simulink model "IEEE14_case"  (R2024b)
settings: Solver=FixedStepAuto  StartTime=0  StopTime=2  FixedStep=1e-7  RelTol=1e-3
values from neighbouring files (symbols this model uses):
  GFL_15_Bva = 0.009    [IEEE14_parameters.m]
  GFL_15_C_bus_pu = 7.179419    [IEEE14_parameters.m]
  GFL_15_f0 = 60    [IEEE14_parameters.m]
  GFL_15_I_id = 691.26967    [IEEE14_parameters.m]
  GFL_15_I_iq = 691.26967    [IEEE14_parameters.m]
  GFL_15_I_od = 45.2207    [IEEE14_parameters.m]
  GFL_15_I_oq = 45.2207    [IEEE14_parameters.m]
  GFL_15_I_pll = 0.78    [IEEE14_parameters.m]
  GFL_15_Kdi = 0.09    [IEEE14_parameters.m]
  GFL_15_Kdo = 0.9    [IEEE14_parameters.m]
  GFL_15_Kqi = 0.09    [IEEE14_parameters.m]
  GFL_15_Kqo = 0.9    [IEEE14_parameters.m]
  GFL_15_Lg_pu = 0.631447    [IEEE14_parameters.m]
  GFL_15_mode = 1    [IEEE14_parameters.m]
  GFL_15_P_id = 3.7166    [IEEE14_parameters.m]
  GFL_15_P_iq = 3.7166    [IEEE14_parameters.m]
  GFL_15_P_od = 0.4798    [IEEE14_parameters.m]
  GFL_15_P_oq = 0.4798    [IEEE14_parameters.m]
  GFL_15_P_pll = 290.42    [IEEE14_parameters.m]
  GFL_15_Qe_ref = 0.2    [IEEE14_parameters.m]
  GFL_15_Rg_pu = 0.024016    [IEEE14_parameters.m]
  GFL_15_Sbase = 1.000000e+4    (= 10000)    [IEEE14_parameters.m]
  GFL_15_Tdi = 0.01    [IEEE14_parameters.m]
  GFL_15_Tdo = 0.2    [IEEE14_parameters.m]
  GFL_15_Tqi = 0.01    [IEEE14_parameters.m]
  GFL_15_Tqo = 0.2    [IEEE14_parameters.m]
  GFL_15_Vbase = 380    [IEEE14_parameters.m]
  GFL_15_Vdc_ref = 1.011475    [IEEE14_parameters.m]
  GFL_15_Vdcbase = 700    [IEEE14_parameters.m]
  GFL_15_vq_ref = 0    [IEEE14_parameters.m]
  GFL_16_Bva = 0.002    [IEEE14_parameters.m]
  GFL_16_C_bus_pu = 7.179419    [IEEE14_parameters.m]
  GFL_16_f0 = 60    [IEEE14_parameters.m]
  GFL_16_I_id = 691.26967    [IEEE14_parameters.m]
  GFL_16_I_iq = 691.26967    [IEEE14_parameters.m]
  GFL_16_I_od = 45.2207    [IEEE14_parameters.m]
  GFL_16_I_oq = 45.2207    [IEEE14_parameters.m]
  GFL_16_I_pll = 0.78    [IEEE14_parameters.m]
  GFL_16_Kdi = 0.05    [IEEE14_parameters.m]
  GFL_16_Kdo = 0.5    [IEEE14_parameters.m]
  GFL_16_Kqi = 0.05    [IEEE14_parameters.m]
  GFL_16_Kqo = 0.5    [IEEE14_parameters.m]
  GFL_16_Lg_pu = 0.631447    [IEEE14_parameters.m]
  GFL_16_mode = 1    [IEEE14_parameters.m]
  GFL_16_P_id = 3.7166    [IEEE14_parameters.m]
  GFL_16_P_iq = 3.7166    [IEEE14_parameters.m]
  GFL_16_P_od = 0.4798    [IEEE14_parameters.m]
  GFL_16_P_oq = 0.4798    [IEEE14_parameters.m]
  GFL_16_P_pll = 290.42    [IEEE14_parameters.m]
  GFL_16_Qe_ref = 0.2    [IEEE14_parameters.m]
  GFL_16_Rg_pu = 0.024016    [IEEE14_parameters.m]
  GFL_16_Sbase = 1.000000e+4    (= 10000)    [IEEE14_parameters.m]
  GFL_16_Tdi = 0.01    [IEEE14_parameters.m]
  GFL_16_Tdo = 0.2    [IEEE14_parameters.m]
  GFL_16_Tqi = 0.01    [IEEE14_parameters.m]
  GFL_16_Tqo = 0.2    [IEEE14_parameters.m]
  GFL_16_Vbase = 380    [IEEE14_parameters.m]
  GFL_16_Vdc_ref = 1.01144    [IEEE14_parameters.m]
  GFL_16_Vdcbase = 700    [IEEE14_parameters.m]
  GFL_16_vq_ref = 0    [IEEE14_parameters.m]
  GFL_17_Bva = 0.002    [IEEE14_parameters.m]
  GFL_17_C_bus_pu = 7.179419    [IEEE14_parameters.m]
  GFL_17_f0 = 60    [IEEE14_parameters.m]
  GFL_17_I_id = 691.26967    [IEEE14_parameters.m]
  GFL_17_I_iq = 691.26967    [IEEE14_parameters.m]
  GFL_17_I_od = 45.2207    [IEEE14_parameters.m]
  GFL_17_I_oq = 45.2207    [IEEE14_parameters.m]
  GFL_17_I_pll = 0.78    [IEEE14_parameters.m]
  GFL_17_Kdi = 0.05    [IEEE14_parameters.m]
  GFL_17_Kdo = 0.5    [IEEE14_parameters.m]
  GFL_17_Kqi = 0.05    [IEEE14_parameters.m]
  GFL_17_Kqo = 0.5    [IEEE14_parameters.m]
  GFL_17_Lg_pu = 0.631447    [IEEE14_parameters.m]
  GFL_17_mode = 1    [IEEE14_parameters.m]
  GFL_17_P_id = 3.7166    [IEEE14_parameters.m]
  GFL_17_P_iq = 3.7166    [IEEE14_parameters.m]
  GFL_17_P_od = 0.4798    [IEEE14_parameters.m]
  GFL_17_P_oq = 0.4798    [IEEE14_parameters.m]
  GFL_17_P_pll = 290.42    [IEEE14_parameters.m]
  GFL_17_Qe_ref = 0.2    [IEEE14_parameters.m]
  GFL_17_Rg_pu = 0.024016    [IEEE14_parameters.m]
  GFL_17_Sbase = 1.000000e+4    (= 10000)    [IEEE14_parameters.m]
  GFL_17_Tdi = 0.01    [IEEE14_parameters.m]
  GFL_17_Tdo = 0.2    [IEEE14_parameters.m]
  GFL_17_Tqi = 0.01    [IEEE14_parameters.m]
  GFL_17_Tqo = 0.2    [IEEE14_parameters.m]
  GFL_17_Vbase = 380    [IEEE14_parameters.m]
  GFL_17_Vdc_ref = 1.011632    [IEEE14_parameters.m]
  GFL_17_Vdcbase = 700    [IEEE14_parameters.m]
  GFL_17_vq_ref = 0    [IEEE14_parameters.m]
  GFL_18_Bva = 0.002    [IEEE14_parameters.m]
  GFL_18_C_bus_pu = 7.179419    [IEEE14_parameters.m]
  GFL_18_f0 = 60    [IEEE14_parameters.m]
  GFL_18_I_id = 691.26967    [IEEE14_parameters.m]
  GFL_18_I_iq = 691.26967    [IEEE14_parameters.m]
  GFL_18_I_od = 45.2207    [IEEE14_parameters.m]
  GFL_18_I_oq = 45.2207    [IEEE14_parameters.m]
  GFL_18_I_pll = 0.78    [IEEE14_parameters.m]
  GFL_18_Kdi = 0.05    [IEEE14_parameters.m]
  GFL_18_Kdo = 0.5    [IEEE14_parameters.m]
  GFL_18_Kqi = 0.05    [IEEE14_parameters.m]
  GFL_18_Kqo = 0.5    [IEEE14_parameters.m]
  GFL_18_Lg_pu = 0.631447    [IEEE14_parameters.m]
  GFL_18_mode = 1    [IEEE14_parameters.m]
  GFL_18_P_id = 3.7166    [IEEE14_parameters.m]
  GFL_18_P_iq = 3.7166    [IEEE14_parameters.m]
  GFL_18_P_od = 0.4798    [IEEE14_parameters.m]
  GFL_18_P_oq = 0.4798    [IEEE14_parameters.m]
  GFL_18_P_pll = 290.42    [IEEE14_parameters.m]
  GFL_18_Qe_ref = 0.2    [IEEE14_parameters.m]
  GFL_18_Rg_pu = 0.024016    [IEEE14_parameters.m]
  GFL_18_Sbase = 1.000000e+4    (= 10000)    [IEEE14_parameters.m]
  GFL_18_Tdi = 0.01    [IEEE14_parameters.m]
  GFL_18_Tdo = 0.2    [IEEE14_parameters.m]
  GFL_18_Tqi = 0.01    [IEEE14_parameters.m]
  GFL_18_Tqo = 0.2    [IEEE14_parameters.m]
  GFL_18_Vbase = 380    [IEEE14_parameters.m]
  GFL_18_Vdc_ref = 1.011572    [IEEE14_parameters.m]
  GFL_18_Vdcbase = 700    [IEEE14_parameters.m]
  GFL_18_vq_ref = 0    [IEEE14_parameters.m]
  ... (+180 more)
(part 5 of 25)

== system IEEE14_case/SG_D_8 ==
  v_d_SG_D_8 : Inport
  v_q_SG_D_8 : Inport  Port=2
  E_fd_SG_D_8 : Integrator  InitialCondition=0.7606400090631968
  Px_1_SG_D_8 : Integrator  InitialCondition=0.0
  Px_2_SG_D_8 : Integrator  InitialCondition=0.0
  Px_3_SG_D_8 : Integrator  InitialCondition=-4.623242258888885e-24
  R_f_SG_D_8 : Integrator  InitialCondition=5.135406689760955
  T_e_SG_D_8_block : Subsystem
  T_m_SG_D_8 : Integrator  InitialCondition=3.269365263487632e-05
  V_f_SG_D_8 : Integrator  InitialCondition=7.606400090631968
  d_E_fd_SG_D_8_block : Subsystem
  d_Px_1_SG_D_8_block : Subsystem
  d_Px_2_SG_D_8_block : Subsystem
  d_Px_3_SG_D_8_block : Subsystem
  d_R_f_SG_D_8_block : Subsystem
  d_T_m_SG_D_8_block : Subsystem
  d_V_f_SG_D_8_block : Subsystem
  d_psi_1d_SG_D_8_block : Subsystem
  d_psi_d_SG_D_8_block : Subsystem
  d_psi_fd_SG_D_8_block : Subsystem
  d_psi_gq_SG_D_8_block : Subsystem
  d_psi_kq_SG_D_8_block : Subsystem
  d_psi_q_SG_D_8_block : Subsystem
  d_theta_SG_D_8_block : Subsystem
  d_w_SG_D_8_block : Subsystem
  i_d_SG_D_8_block : Subsystem
  i_q_SG_D_8_block : Subsystem
  psi_1d_SG_D_8 : Integrator  InitialCondition=1.08133264662511
  psi_d_SG_D_8 : Integrator  InitialCondition=1.0900000152078642
  psi_fd_SG_D_8 : Integrator  InitialCondition=1.0376491089680278
  psi_gq_SG_D_8 : Integrator  InitialCondition=3.0249198689621347e-05
  psi_kq_SG_D_8 : Integrator  InitialCondition=-4.726437295253334e-05
  psi_q_SG_D_8 : Integrator  InitialCondition=-4.9154947870634654e-05
  theta_SG_D_8 : Integrator  InitialCondition=-0.18629255619094007
  theta_SG_D_8_out_block : Subsystem
  w_SG_D_8 : Integrator  InitialCondition=376.99111843077515
  w_SG_D_8_out_block : Subsystem
  i_d_SG_D_8 : Outport
  i_q_SG_D_8 : Outport  Port=2
  T_e_SG_D_8 : Outport  Port=3
  w_SG_D_8_out : Outport  Port=4
  theta_SG_D_8_out : Outport  Port=5
  wires:
  d_T_m_SG_D_8_block/1(Blockout_d_T_m_SG_D_8_65767) -> T_m_SG_D_8/1
  T_e_SG_D_8_block/1(Blockout_T_e_SG_D_8_36eef) -> T_e_SG_D_8/1
  theta_SG_D_8/1 -> d_psi_d_SG_D_8_block/5(State_theta_SG_D_8_aea71), d_psi_q_SG_D_8_block/5(State_theta_SG_D_8_01782), i_d_SG_D_8_block/4(State_theta_SG_D_8_641e8), i_d_SG_D_8_block/8(State_theta_SG_D_8_bcf58), d_psi_q_SG_D_8_block/7(State_theta_SG_D_8_5a3fa), i_q_SG_D_8_block/8(State_theta_SG_D_8_83255), d_psi_d_SG_D_8_block/7(State_theta_SG_D_8_9f713), theta_SG_D_8_out_block/1(State_theta_SG_D_8_cdb63), i_q_SG_D_8_block/4(State_theta_SG_D_8_df609)
  w_SG_D_8/1 -> d_psi_d_SG_D_8_block/9(State_w_SG_D_8_03911), d_psi_q_SG_D_8_block/9(State_w_SG_D_8_716c2), d_w_SG_D_8_block/1(State_w_SG_D_8_a443d), d_V_f_SG_D_8_block/8(State_w_SG_D_8_6dc7e), d_T_m_SG_D_8_block/1(State_w_SG_D_8_04413), d_theta_SG_D_8_block/1(State_w_SG_D_8_7874c), d_V_f_SG_D_8_block/13(State_w_SG_D_8_608f6), d_Px_2_SG_D_8_block/4(State_w_SG_D_8_213d1), d_Px_3_SG_D_8_block/6(State_w_SG_D_8_deb3f), w_SG_D_8_out_block/1(State_w_SG_D_8_62717), d_Px_1_SG_D_8_block/2(State_w_SG_D_8_14513)
  d_Px_2_SG_D_8_block/1(Blockout_d_Px_2_SG_D_8_ad385) -> Px_2_SG_D_8/1
  E_fd_SG_D_8/1 -> d_V_f_SG_D_8_block/1(State_E_fd_SG_D_8_0863f), d_E_fd_SG_D_8_block/1(State_E_fd_SG_D_8_6df86), d_R_f_SG_D_8_block/1(State_E_fd_SG_D_8_d418e), d_psi_fd_SG_D_8_block/1(State_E_fd_SG_D_8_e02cf)
  R_f_SG_D_8/1 -> d_V_f_SG_D_8_block/2(State_R_f_SG_D_8_6736f), d_R_f_SG_D_8_block/2(State_R_f_SG_D_8_19ab3)
  d_R_f_SG_D_8_block/1(Blockout_d_R_f_SG_D_8_431b8) -> R_f_SG_D_8/1
  w_SG_D_8_out_block/1(Blockout_w_SG_D_8_out_d72e6) -> w_SG_D_8_out/1
  d_Px_1_SG_D_8_block/1(Blockout_d_Px_1_SG_D_8_010b5) -> Px_1_SG_D_8/1
  d_theta_SG_D_8_block/1(Blockout_d_theta_SG_D_8_7fdd6) -> theta_SG_D_8/1
  d_Px_3_SG_D_8_block/1(Blockout_d_Px_3_SG_D_8_b7d57) -> Px_3_SG_D_8/1
  psi_gq_SG_D_8/1 -> d_psi_q_SG_D_8_block/1(State_psi_gq_SG_D_8_a7fd3), d_psi_gq_SG_D_8_block/1(State_psi_gq_SG_D_8_21c0a), d_psi_gq_SG_D_8_block/2(State_psi_gq_SG_D_8_953e4), d_psi_gq_SG_D_8_block/7(State_psi_gq_SG_D_8_869cf), d_psi_kq_SG_D_8_block/1(State_psi_gq_SG_D_8_46c2d), d_psi_kq_SG_D_8_block/3(State_psi_gq_SG_D_8_4cdf1), d_w_SG_D_8_block/4(State_psi_gq_SG_D_8_6cde6), i_d_SG_D_8_block/1(State_psi_gq_SG_D_8_6ad23), i_q_SG_D_8_block/1(State_psi_gq_SG_D_8_d57d0), d_V_f_SG_D_8_block/9(State_psi_gq_SG_D_8_341db), T_e_SG_D_8_block/2(State_psi_gq_SG_D_8_ece9e), d_psi_gq_SG_D_8_block/4(State_psi_gq_SG_D_8_d7d68)
  T_m_SG_D_8/1 -> d_T_m_SG_D_8_block/2(State_T_m_SG_D_8_6d384), d_w_SG_D_8_block/2(State_T_m_SG_D_8_49ad0)
  psi_q_SG_D_8/1 -> d_psi_d_SG_D_8_block/8(State_psi_q_SG_D_8_b70d1), d_psi_q_SG_D_8_block/3(State_psi_q_SG_D_8_e0430), d_psi_gq_SG_D_8_block/6(State_psi_q_SG_D_8_5d8c1), d_psi_gq_SG_D_8_block/9(State_psi_q_SG_D_8_ecb47), d_psi_kq_SG_D_8_block/5(State_psi_q_SG_D_8_6f170), d_w_SG_D_8_block/6(State_psi_q_SG_D_8_202ce), d_w_SG_D_8_block/7(State_psi_q_SG_D_8_9c5c1), d_V_f_SG_D_8_block/11(State_psi_q_SG_D_8_d5d6d), i_q_SG_D_8_block/3(State_psi_q_SG_D_8_a812b), i_d_SG_D_8_block/3(State_psi_q_SG_D_8_2ca29), T_e_SG_D_8_block/4(State_psi_q_SG_D_8_1c36c), d_V_f_SG_D_8_block/7(State_psi_q_SG_D_8_e1efb), T_e_SG_D_8_block/5(State_psi_q_SG_D_8_67075)
  Px_2_SG_D_8/1 -> d_Px_2_SG_D_8_block/1(State_Px_2_SG_D_8_4dc99), d_Px_3_SG_D_8_block/2(State_Px_2_SG_D_8_f1029), d_Px_3_SG_D_8_block/3(State_Px_2_SG_D_8_bb5ac)
  Px_3_SG_D_8/1 -> d_Px_3_SG_D_8_block/1(State_Px_3_SG_D_8_df285), d_V_f_SG_D_8_block/3(State_Px_3_SG_D_8_1b788)
  v_d_SG_D_8/1 -> d_psi_d_SG_D_8_block/4(Input_v_d_SG_D_8_41885), d_psi_q_SG_D_8_block/4(Input_v_d_SG_D_8_c09e8)
  d_psi_gq_SG_D_8_block/1(Blockout_d_psi_gq_SG_D_8_03a58) -> psi_gq_SG_D_8/1
  v_q_SG_D_8/1 -> d_psi_d_SG_D_8_block/6(Input_v_q_SG_D_8_e5b6f), d_psi_q_SG_D_8_block/6(Input_v_q_SG_D_8_1ed15)
  d_psi_1d_SG_D_8_block/1(Blockout_d_psi_1d_SG_D_8_20ff0) -> psi_1d_SG_D_8/1
  psi_fd_SG_D_8/1 -> d_psi_fd_SG_D_8_block/2(State_psi_fd_SG_D_8_39b4d), d_psi_fd_SG_D_8_block/4(State_psi_fd_SG_D_8_1b7c8), d_psi_fd_SG_D_8_block/7(State_psi_fd_SG_D_8_ed057), d_psi_fd_SG_D_8_block/10(State_psi_fd_SG_D_8_f6f0f), d_psi_d_SG_D_8_block/3(State_psi_fd_SG_D_8_f0d2e), d_psi_1d_SG_D_8_block/5(State_psi_fd_SG_D_8_c65e7), d_w_SG_D_8_block/10(State_psi_fd_SG_D_8_93d32), d_psi_1d_SG_D_8_block/2(State_psi_fd_SG_D_8_4604f), i_d_SG_D_8_block/7(State_psi_fd_SG_D_8_06311), i_q_SG_D_8_block/7(State_psi_fd_SG_D_8_e7c26), d_V_f_SG_D_8_block/6(State_psi_fd_SG_D_8_8705e), T_e_SG_D_8_block/8(State_psi_fd_SG_D_8_0a0bc)
  psi_1d_SG_D_8/1 -> d_psi_fd_SG_D_8_block/3(State_psi_1d_SG_D_8_31c78), d_psi_fd_SG_D_8_block/5(State_psi_1d_SG_D_8_9e1bf), d_psi_fd_SG_D_8_block/8(State_psi_1d_SG_D_8_5095e), d_psi_d_SG_D_8_block/1(State_psi_1d_SG_D_8_3a1ac), d_psi_1d_SG_D_8_block/3(State_psi_1d_SG_D_8_0fd5c), i_d_SG_D_8_block/5(State_psi_1d_SG_D_8_b3820), i_q_SG_D_8_block/5(State_psi_1d_SG_D_8_47e6f), T_e_SG_D_8_block/6(State_psi_1d_SG_D_8_d92c8), d_V_f_SG_D_8_block/4(State_psi_1d_SG_D_8_0200e), d_psi_1d_SG_D_8_block/1(State_psi_1d_SG_D_8_961b1), d_w_SG_D_8_block/8(State_psi_1d_SG_D_8_25d54)
  psi_d_SG_D_8/1 -> d_psi_fd_SG_D_8_block/6(State_psi_d_SG_D_8_43284), d_psi_fd_SG_D_8_block/9(State_psi_d_SG_D_8_8f483), d_psi_d_SG_D_8_block/2(State_psi_d_SG_D_8_aedd8), d_psi_1d_SG_D_8_block/4(State_psi_d_SG_D_8_df1ee), d_w_SG_D_8_block/3(State_psi_d_SG_D_8_19a89), d_w_SG_D_8_block/9(State_psi_d_SG_D_8_5f3fa), d_V_f_SG_D_8_block/5(State_psi_d_SG_D_8_c5413), d_V_f_SG_D_8_block/12(State_psi_d_SG_D_8_14bfc), i_d_SG_D_8_block/6(State_psi_d_SG_D_8_f7e33), i_q_SG_D_8_block/6(State_psi_d_SG_D_8_17299), T_e_SG_D_8_block/7(State_psi_d_SG_D_8_41989), d_psi_q_SG_D_8_block/8(State_psi_d_SG_D_8_332cc), T_e_SG_D_8_block/1(State_psi_d_SG_D_8_8bce2)
  psi_kq_SG_D_8/1 -> d_psi_q_SG_D_8_block/2(State_psi_kq_SG_D_8_644c1), d_psi_gq_SG_D_8_block/3(State_psi_kq_SG_D_8_6a8ed), d_psi_gq_SG_D_8_block/5(State_psi_kq_SG_D_8_1ecc5), d_psi_kq_SG_D_8_block/2(State_psi_kq_SG_D_8_36a8a), d_psi_gq_SG_D_8_block/8(State_psi_kq_SG_D_8_7be32), d_psi_kq_SG_D_8_block/4(State_psi_kq_SG_D_8_90e06), i_d_SG_D_8_block/2(State_psi_kq_SG_D_8_4cd34), d_w_SG_D_8_block/5(State_psi_kq_SG_D_8_f145c), i_q_SG_D_8_block/2(State_psi_kq_SG_D_8_4aaa9), d_V_f_SG_D_8_block/10(State_psi_kq_SG_D_8_85c57), T_e_SG_D_8_block/3(State_psi_kq_SG_D_8_39808)
  Px_1_SG_D_8/1 -> d_Px_1_SG_D_8_block/1(State_Px_1_SG_D_8_6e138), d_Px_3_SG_D_8_block/4(State_Px_1_SG_D_8_7f9bd), d_Px_2_SG_D_8_block/3(State_Px_1_SG_D_8_35ac2), d_Px_2_SG_D_8_block/2(State_Px_1_SG_D_8_d499c), d_Px_3_SG_D_8_block/5(State_Px_1_SG_D_8_8b47e)
  d_w_SG_D_8_block/1(Blockout_d_w_SG_D_8_91fe0) -> w_SG_D_8/1
  d_psi_kq_SG_D_8_block/1(Blockout_d_psi_kq_SG_D_8_f1e70) -> psi_kq_SG_D_8/1
  d_V_f_SG_D_8_block/1(Blockout_d_V_f_SG_D_8_302ea) -> V_f_SG_D_8/1
  d_psi_q_SG_D_8_block/1(Blockout_d_psi_q_SG_D_8_90d0e) -> psi_q_SG_D_8/1
  d_psi_d_SG_D_8_block/1(Blockout_d_psi_d_SG_D_8_dc023) -> psi_d_SG_D_8/1
  i_q_SG_D_8_block/1(Blockout_i_q_SG_D_8_09699) -> i_q_SG_D_8/1
  i_d_SG_D_8_block/1(Blockout_i_d_SG_D_8_0f0f6) -> i_d_SG_D_8/1
  theta_SG_D_8_out_block/1(Blockout_theta_SG_D_8_out_2e6e5) -> theta_SG_D_8_out/1
  V_f_SG_D_8/1 -> d_V_f_SG_D_8_block/14(State_V_f_SG_D_8_f18fe), d_E_fd_SG_D_8_block/2(State_V_f_SG_D_8_2f3e7)
  d_E_fd_SG_D_8_block/1(Blockout_d_E_fd_SG_D_8_bd076) -> E_fd_SG_D_8/1
  d_psi_fd_SG_D_8_block/1(Blockout_d_psi_fd_SG_D_8_d8ca3) -> psi_fd_SG_D_8/1

== system IEEE14_case/Subsystem ==
  In1 : Inport
  In2 : Inport  Port=2
  In3 : Inport  Port=3
  In4 : Inport  Port=4
  Add : Sum
  Product : Product
  Product1 : Product
  Out1 : Outport
  wires:
  Product/1 -> Add/1
  In1/1 -> Product/1
  In3/1 -> Product1/1
  In2/1 -> Product/2
  Add/1 -> Out1/1
  Product1/1 -> Add/2
  In4/1 -> Product1/2

== system IEEE14_case/Subsystem1 ==
  In1 : Inport
  In2 : Inport  Port=2
  In3 : Inport  Port=3
  In4 : Inport  Port=4
  Add1 : Sum  Inputs=+-
  Product2 : Product
  Product3 : Product
  Out1 : Outport
  wires:
  In4/1 -> Product3/2
  Product3/1 -> Add1/2
  Product2/1 -> Add1/1
  In3/1 -> Product3/1
  In1/1 -> Product2/1
  Add1/1 -> Out1/1
  In2/1 -> Product2/2

== system IEEE14_case/AC_1/d_id_line_10_11_block ==
  note: d_id_line_10_11 in case14gfl
      | $376.991118430775\,\mathrm{iq}_{\mathrm{line},10,11}-161.046083548941\,\mathrm{id}_{\mathrm{line},10,11}+1962.77981168728\,\mathrm{vd}_{\mathrm{bus},10}-1962.77981168728\,\mathrm{vd}_{\mathrm{bus},11}$
      | Automatically generated on 2025-10-09 21:39:46 .
  State_id_line_10_11_cd03d : Inport
  State_iq_line_10_11_98837 : Inport  Port=2
  State_vd_bus_10_b9381 : Inport  Port=3
  State_vd_bus_11_0464d : Inport  Port=4
  Add_044af : Sum
  Add_952f4 : Sum
  Constant_-161.046083548941_02036 : Constant  Value=-161.046083548941
  Constant_1962.77981168728_222ef : Constant  Value=1962.77981168728
  Constant_1962.77981168728_ae5a8 : Constant  Value=1962.77981168728
  Constant_376.991118430775_6ba22 : Constant  Value=376.991118430775
  Product_7b56a : Product
  Product_7fb11 : Product
  Product_aa4a9 : Product
  Product_fe1f1 : Product
  Subtract_21330 : Sum  Inputs=+-
  Blockout_d_id_line_10_11_2eb24 : Outport
  wires:
  Constant_-161.046083548941_02036/1 -> Product_7b56a/1
  Subtract_21330/1 -> Blockout_d_id_line_10_11_2eb24/1
  State_id_line_10_11_cd03d/1 -> Product_7b56a/2
  Constant_376.991118430775_6ba22/1 -> Product_aa4a9/1
  Product_aa4a9/1 -> Add_044af/2
  Product_7fb11/1 -> Add_952f4/2
  Constant_1962.77981168728_222ef/1 -> Product_7fb11/1
  State_iq_line_10_11_98837/1 -> Product_aa4a9/2
  Product_7b56a/1 -> Add_044af/1
  State_vd_bus_10_b9381/1 -> Product_7fb11/2
  Add_044af/1 -> Add_952f4/1
  Product_fe1f1/1 -> Subtract_21330/2
  Constant_1962.77981168728_ae5a8/1 -> Product_fe1f1/1
  State_vd_bus_11_0464d/1 -> Product_fe1f1/2
  Add_952f4/1 -> Subtract_21330/1

== system IEEE14_case/AC_1/d_id_line_11_15_block ==
  note: d_id_line_11_15 in case14gfl
      | $376.991118430775\,\mathrm{iq}_{\mathrm{line},11,15}-32.3135244369236\,\mathrm{id}_{\mathrm{line},11,15}+538.558740615393\,\mathrm{vd}_{\mathrm{bus},11}-538.558740615393\,\mathrm{vd}_{\mathrm{bus},15}$
      | Automatically generated on 2025-10-09 21:39:53 .
  State_id_line_11_15_bc21e : Inport
  State_iq_line_11_15_e6608 : Inport  Port=2
  State_vd_bus_11_d33d1 : Inport  Port=3
  State_vd_bus_15_a703b : Inport  Port=4
  Add_9e7fa : Sum
  Add_ec072 : Sum
  Constant_-32.3135244369236_ce476 : Constant  Value=-32.3135244369236
  Constant_376.991118430775_cd329 : Constant  Value=376.991118430775
  Constant_538.558740615393_1f99f : Constant  Value=538.558740615393
  Constant_538.558740615393_64059 : Constant  Value=538.558740615393
  Product_5d9cb : Product
  Product_5fd59 : Product
  Product_c3b90 : Product
  Product_c9bc5 : Product
  Subtract_ad8a8 : Sum  Inputs=+-
  Blockout_d_id_line_11_15_7b448 : Outport
  wires:
  Constant_-32.3135244369236_ce476/1 -> Product_5d9cb/1
  Product_5d9cb/1 -> Add_ec072/1
  State_id_line_11_15_bc21e/1 -> Product_5d9cb/2
  Constant_376.991118430775_cd329/1 -> Product_c9bc5/1
  Product_c9bc5/1 -> Add_ec072/2
  State_iq_line_11_15_e6608/1 -> Product_c9bc5/2
  State_vd_bus_11_d33d1/1 -> Product_c3b90/2
  Product_c3b90/1 -> Add_9e7fa/2
  Constant_538.558740615393_64059/1 -> Product_c3b90/1
  Add_ec072/1 -> Add_9e7fa/1
  Product_5fd59/1 -> Subtract_ad8a8/2
  Constant_538.558740615393_1f99f/1 -> Product_5fd59/1
  Add_9e7fa/1 -> Subtract_ad8a8/1
  State_vd_bus_15_a703b/1 -> Product_5fd59/2
  Subtract_ad8a8/1 -> Blockout_d_id_line_11_15_7b448/1

== system IEEE14_case/AC_1/d_id_line_12_13_block ==
  note: d_id_line_12_13 in case14gfl
      | $376.991118430775\,\mathrm{iq}_{\mathrm{line},12,13}-416.674394055067\,\mathrm{id}_{\mathrm{line},12,13}+1886.08724450058\,\mathrm{vd}_{\mathrm{bus},12}-1886.08724450058\,\mathrm{vd}_{\mathrm{bus},13}$
      | Automatically generated on 2025-10-09 21:39:48 .
  State_id_line_12_13_dd6c1 : Inport
  State_iq_line_12_13_bd70b : Inport  Port=2
  State_vd_bus_12_5b3a8 : Inport  Port=3
  State_vd_bus_13_1a95e : Inport  Port=4
  Add_3f260 : Sum
  Add_fb038 : Sum
  Constant_-416.674394055067_9eb27 : Constant  Value=-416.674394055067
  Constant_1886.08724450058_572fc : Constant  Value=1886.08724450058
  Constant_1886.08724450058_d19a4 : Constant  Value=1886.08724450058
  Constant_376.991118430775_8657a : Constant  Value=376.991118430775
  Product_08de4 : Product
  Product_09161 : Product
  Product_3ee40 : Product
  Product_c6c0f : Product
  Subtract_69e56 : Sum  Inputs=+-
  Blockout_d_id_line_12_13_a63f9 : Outport
  wires:
  State_iq_line_12_13_bd70b/1 -> Product_3ee40/2
  Constant_-416.674394055067_9eb27/1 -> Product_08de4/1
  Constant_376.991118430775_8657a/1 -> Product_3ee40/1
  Product_3ee40/1 -> Add_fb038/2
  State_id_line_12_13_dd6c1/1 -> Product_08de4/2
  Product_08de4/1 -> Add_fb038/1
  Constant_1886.08724450058_d19a4/1 -> Product_09161/1
  State_vd_bus_12_5b3a8/1 -> Product_09161/2
  Add_fb038/1 -> Add_3f260/1
  Product_09161/1 -> Add_3f260/2
  Product_c6c0f/1 -> Subtract_69e56/2
  Constant_1886.08724450058_572fc/1 -> Product_c6c0f/1
  State_vd_bus_13_1a95e/1 -> Product_c6c0f/2
  Add_3f260/1 -> Subtract_69e56/1
  Subtract_69e56/1 -> Blockout_d_id_line_12_13_a63f9/1

== system IEEE14_case/AC_1/d_id_line_12_16_block ==
  note: d_id_line_12_16 in case14gfl
      | $376.991118430775\,\mathrm{iq}_{\mathrm{line},12,16}-32.3135244369236\,\mathrm{id}_{\mathrm{line},12,16}+538.558740615393\,\mathrm{vd}_{\mathrm{bus},12}-538.558740615393\,\mathrm{vd}_{\mathrm{bus},16}$
      | Automatically generated on 2025-10-09 21:39:55 .
  State_id_line_12_16_7c285 : Inport
  State_iq_line_12_16_b3649 : Inport  Port=2
  State_vd_bus_12_7f21e : Inport  Port=3
  State_vd_bus_16_b2ca7 : Inport  Port=4
  Add_71088 : Sum
  Add_cefde : Sum
  Constant_-32.3135244369236_989f2 : Constant  Value=-32.3135244369236
  Constant_376.991118430775_4638c : Constant  Value=376.991118430775
  Constant_538.558740615393_259c1 : Constant  Value=538.558740615393
  Constant_538.558740615393_4455a : Constant  Value=538.558740615393
  Product_4a5f5 : Product
  Product_8747e : Product
  Product_c16a2 : Product
  Product_f3dc0 : Product
  Subtract_95055 : Sum  Inputs=+-
  Blockout_d_id_line_12_16_c0fbf : Outport
  wires:
  State_id_line_12_16_7c285/1 -> Product_8747e/2
  Constant_-32.3135244369236_989f2/1 -> Product_8747e/1
  Constant_376.991118430775_4638c/1 -> Product_4a5f5/1
  Product_4a5f5/1 -> Add_71088/2
  Product_c16a2/1 -> Add_cefde/2
  Constant_538.558740615393_259c1/1 -> Product_c16a2/1
  State_iq_line_12_16_b3649/1 -> Product_4a5f5/2
  Product_8747e/1 -> Add_71088/1
  State_vd_bus_12_7f21e/1 -> Product_c16a2/2
  Add_71088/1 -> Add_cefde/1
  Product_f3dc0/1 -> Subtract_95055/2
  Constant_538.558740615393_4455a/1 -> Product_f3dc0/1
  State_vd_bus_16_b2ca7/1 -> Product_f3dc0/2
  Add_cefde/1 -> Subtract_95055/1
  Subtract_95055/1 -> Blockout_d_id_line_12_16_c0fbf/1

== system IEEE14_case/AC_1/d_id_line_13_14_block ==
  note: d_id_line_13_14 in case14gfl
      | $376.991118430775\,\mathrm{iq}_{\mathrm{line},13,14}-185.159162902627\,\mathrm{id}_{\mathrm{line},13,14}+1083.24555609096\,\mathrm{vd}_{\mathrm{bus},13}-1083.24555609096\,\mathrm{vd}_{\mathrm{bus},14}$
      | Automatically generated on 2025-10-09 21:39:50 .
  State_id_line_13_14_79a4b : Inport
  State_iq_line_13_14_4cdf7 : Inport  Port=2
  State_vd_bus_13_a4a43 : Inport  Port=3
  State_vd_bus_14_db328 : Inport  Port=4
  Add_2b3ae : Sum
  Add_92208 : Sum
  Constant_-185.159162902627_131b7 : Constant  Value=-185.159162902627
  Constant_1083.24555609096_5a0e7 : Constant  Value=1083.24555609096
  Constant_1083.24555609096_8e61e : Constant  Value=1083.24555609096
  Constant_376.991118430775_13321 : Constant  Value=376.991118430775
  Product_45268 : Product
  Product_c11f5 : Product
  Product_da29c : Product
  Product_f0334 : Product
  Subtract_95086 : Sum  Inputs=+-
  Blockout_d_id_line_13_14_fab77 : Outport
  wires:
  Constant_-185.159162902627_131b7/1 -> Product_45268/1
  Product_45268/1 -> Add_2b3ae/1
  Subtract_95086/1 -> Blockout_d_id_line_13_14_fab77/1
  State_id_line_13_14_79a4b/1 -> Product_45268/2
  Constant_376.991118430775_13321/1 -> Product_c11f5/1
  Product_c11f5/1 -> Add_2b3ae/2
  State_iq_line_13_14_4cdf7/1 -> Product_c11f5/2
  Product_f0334/1 -> Add_92208/2
  Constant_1083.24555609096_8e61e/1 -> Product_f0334/1
  State_vd_bus_13_a4a43/1 -> Product_f0334/2
  Add_2b3ae/1 -> Add_92208/1
  Constant_1083.24555609096_5a0e7/1 -> Product_da29c/1
  State_vd_bus_14_db328/1 -> Product_da29c/2
  Add_92208/1 -> Subtract_95086/1
  Product_da29c/1 -> Subtract_95086/2

== system IEEE14_case/AC_1/d_id_line_13_17_block ==
  note: d_id_line_13_17 in case14gfl
      | $376.991118430775\,\mathrm{iq}_{\mathrm{line},13,17}-32.3135244369236\,\mathrm{id}_{\mathrm{line},13,17}+538.558740615393\,\mathrm{vd}_{\mathrm{bus},13}-538.558740615393\,\mathrm{vd}_{\mathrm{bus},17}$
      | Automatically generated on 2025-10-09 21:39:57 .
  State_id_line_13_17_86061 : Inport
  State_iq_line_13_17_a0741 : Inport  Port=2
  State_vd_bus_13_e5c14 : Inport  Port=3
  State_vd_bus_17_94433 : Inport  Port=4
  Add_85017 : Sum
  Add_b41df : Sum
  Constant_-32.3135244369236_c0773 : Constant  Value=-32.3135244369236
  Constant_376.991118430775_c840a : Constant  Value=376.991118430775
  Constant_538.558740615393_15349 : Constant  Value=538.558740615393
  Constant_538.558740615393_4ce18 : Constant  Value=538.558740615393
  Product_17a6a : Product
  Product_257da : Product
  Product_a0416 : Product
  Product_e7a08 : Product
  Subtract_3675c : Sum  Inputs=+-
  Blockout_d_id_line_13_17_24730 : Outport
  wires:
  State_iq_line_13_17_a0741/1 -> Product_a0416/2
  Constant_-32.3135244369236_c0773/1 -> Product_e7a08/1
  Constant_376.991118430775_c840a/1 -> Product_a0416/1
  Product_a0416/1 -> Add_85017/2
  State_id_line_13_17_86061/1 -> Product_e7a08/2
  Product_e7a08/1 -> Add_85017/1
  Constant_538.558740615393_4ce18/1 -> Product_257da/1
  State_vd_bus_13_e5c14/1 -> Product_257da/2
  Add_85017/1 -> Add_b41df/1
  Product_257da/1 -> Add_b41df/2
  Product_17a6a/1 -> Subtract_3675c/2
  Constant_538.558740615393_15349/1 -> Product_17a6a/1
  State_vd_bus_17_94433/1 -> Product_17a6a/2
  Add_b41df/1 -> Subtract_3675c/1
  Subtract_3675c/1 -> Blockout_d_id_line_13_17_24730/1

== system IEEE14_case/AC_1/d_id_line_14_18_block ==
  note: d_id_line_14_18 in case14gfl
      | $376.991118430775\,\mathrm{iq}_{\mathrm{line},14,18}-32.3135244369236\,\mathrm{id}_{\mathrm{line},14,18}+538.558740615393\,\mathrm{vd}_{\mathrm{bus},14}-538.558740615393\,\mathrm{vd}_{\mathrm{bus},18}$
      | Automatically generated on 2025-10-09 21:40:00 .
  State_id_line_14_18_fb6d6 : Inport
  State_iq_line_14_18_a74d0 : Inport  Port=2
  State_vd_bus_14_f98b2 : Inport  Port=3
  State_vd_bus_18_b444f : Inport  Port=4
  Add_15b48 : Sum
  Add_7e766 : Sum
  Constant_-32.3135244369236_f6a71 : Constant  Value=-32.3135244369236
  Constant_376.991118430775_92094 : Constant  Value=376.991118430775
  Constant_538.558740615393_c6265 : Constant  Value=538.558740615393
  Constant_538.558740615393_d688d : Constant  Value=538.558740615393
  Product_0bcce : Product
  Product_44810 : Product
  Product_4ac6d : Product
  Product_99de6 : Product
  Subtract_b7c2c : Sum  Inputs=+-
  Blockout_d_id_line_14_18_3e263 : Outport
  wires:
  Constant_-32.3135244369236_f6a71/1 -> Product_99de6/1
  Product_99de6/1 -> Add_15b48/1
  State_id_line_14_18_fb6d6/1 -> Product_99de6/2
  Constant_376.991118430775_92094/1 -> Product_4ac6d/1
  Product_4ac6d/1 -> Add_15b48/2
  State_iq_line_14_18_a74d0/1 -> Product_4ac6d/2
  Product_0bcce/1 -> Add_7e766/2
  Constant_538.558740615393_c6265/1 -> Product_0bcce/1
  State_vd_bus_14_f98b2/1 -> Product_0bcce/2
  Add_15b48/1 -> Add_7e766/1
  Constant_538.558740615393_d688d/1 -> Product_44810/1
  State_vd_bus_18_b444f/1 -> Product_44810/2
  Add_7e766/1 -> Subtract_b7c2c/1
  Product_44810/1 -> Subtract_b7c2c/2
  Subtract_b7c2c/1 -> Blockout_d_id_line_14_18_3e263/1

== system IEEE14_case/AC_1/d_id_line_1_2_block ==
  note: d_id_line_1_2 in case14gfl
      | $376.991118430775\,\mathrm{iq}_{\mathrm{line},1,2}-123.476218948596\,\mathrm{id}_{\mathrm{line},1,2}+6371.32192717213\,\mathrm{vd}_{\mathrm{bus},1}-6371.32192717213\,\mathrm{vd}_{\mathrm{bus},2}$
      | Automatically generated on 2025-10-09 21:39:11 .
  State_id_line_1_2_4e64f : Inport
  State_iq_line_1_2_aada7 : Inport  Port=2
  State_vd_bus_1_70d37 : Inport  Port=3
  State_vd_bus_2_c09e1 : Inport  Port=4
  Add_a1930 : Sum
  Add_e754f : Sum
  Constant_-123.476218948596_5bf1b : Constant  Value=-123.476218948596
  Constant_376.991118430775_40784 : Constant  Value=376.991118430775
  Constant_6371.32192717213_38569 : Constant  Value=6371.32192717213
  Constant_6371.32192717213_e91b8 : Constant  Value=6371.32192717213
  Product_2be0d : Product
  Product_33e9b : Product
  Product_7e726 : Product
  Product_85465 : Product
  Subtract_08e95 : Sum  Inputs=+-
  Blockout_d_id_line_1_2_e6d8f : Outport
  wires:
  Constant_-123.476218948596_5bf1b/1 -> Product_2be0d/1
  Product_2be0d/1 -> Add_e754f/1
  State_id_line_1_2_4e64f/1 -> Product_2be0d/2
  Add_a1930/1 -> Subtract_08e95/1
  Constant_376.991118430775_40784/1 -> Product_33e9b/1
  Product_33e9b/1 -> Add_e754f/2
  State_iq_line_1_2_aada7/1 -> Product_33e9b/2
  Product_7e726/1 -> Add_a1930/2
  Constant_6371.32192717213_38569/1 -> Product_7e726/1
  Subtract_08e95/1 -> Blockout_d_id_line_1_2_e6d8f/1
  State_vd_bus_1_70d37/1 -> Product_7e726/2
  Add_e754f/1 -> Add_a1930/1
  Product_85465/1 -> Subtract_08e95/2
  Constant_6371.32192717213_e91b8/1 -> Product_85465/1
  State_vd_bus_2_c09e1/1 -> Product_85465/2

== system IEEE14_case/AC_1/d_id_line_1_5_block ==
  note: d_id_line_1_5 in case14gfl
      | $376.991118430775\,\mathrm{iq}_{\mathrm{line},1,5}-91.3236644943274\,\mathrm{id}_{\mathrm{line},1,5}+1690.23994992277\,\mathrm{vd}_{\mathrm{bus},1}-1690.23994992277\,\mathrm{vd}_{\mathrm{bus},5}$
      | Automatically generated on 2025-10-09 21:39:13 .
  State_id_line_1_5_7d5d3 : Inport
  State_iq_line_1_5_368c4 : Inport  Port=2
  State_vd_bus_1_768e4 : Inport  Port=3
  State_vd_bus_5_58650 : Inport  Port=4
  Add_8fb67 : Sum
  Add_b211a : Sum
  Constant_-91.3236644943274_4a822 : Constant  Value=-91.3236644943274
  Constant_1690.23994992277_5f559 : Constant  Value=1690.23994992277
  Constant_1690.23994992277_87596 : Constant  Value=1690.23994992277
  Constant_376.991118430775_d449f : Constant  Value=376.991118430775
  Product_0e523 : Product
  Product_275fb : Product
  Product_4af4f : Product
  Product_fdc0d : Product
  Subtract_4765f : Sum  Inputs=+-
  Blockout_d_id_line_1_5_95dd5 : Outport
  wires:
  Constant_-91.3236644943274_4a822/1 -> Product_0e523/1
  State_id_line_1_5_7d5d3/1 -> Product_0e523/2
  Constant_376.991118430775_d449f/1 -> Product_275fb/1
  Product_275fb/1 -> Add_b211a/2
  State_iq_line_1_5_368c4/1 -> Product_275fb/2
  Product_0e523/1 -> Add_b211a/1
  Constant_1690.23994992277_5f559/1 -> Product_4af4f/1
  State_vd_bus_1_768e4/1 -> Product_4af4f/2
  Add_b211a/1 -> Add_8fb67/1
  Product_4af4f/1 -> Add_8fb67/2
  Product_fdc0d/1 -> Subtract_4765f/2
  Constant_1690.23994992277_87596/1 -> Product_fdc0d/1
  State_vd_bus_5_58650/1 -> Product_fdc0d/2
  Add_8fb67/1 -> Subtract_4765f/1
  Subtract_4765f/1 -> Blockout_d_id_line_1_5_95dd5/1

== system IEEE14_case/AC_1/d_id_line_2_3_block ==
  note: d_id_line_2_3 in case14gfl
      | $376.991118430775\,\mathrm{iq}_{\mathrm{line},2,3}-89.482308708704\,\mathrm{id}_{\mathrm{line},2,3}+1904.28407552041\,\mathrm{vd}_{\mathrm{bus},2}-1904.28407552041\,\mathrm{vd}_{\mathrm{bus},3}$
      | Automatically generated on 2025-10-09 21:39:15 .
  State_id_line_2_3_bbe6e : Inport
  State_iq_line_2_3_6cbab : Inport  Port=2
  State_vd_bus_2_5855d : Inport  Port=3
  State_vd_bus_3_a3e95 : Inport  Port=4
  Add_6ef66 : Sum
  Add_ba6b5 : Sum
  Constant_-89.482308708704_658cd : Constant  Value=-89.482308708704
  Constant_1904.28407552041_4ffae : Constant  Value=1904.28407552041
  Constant_1904.28407552041_cec53 : Constant  Value=1904.28407552041
  Constant_376.991118430775_7f626 : Constant  Value=376.991118430775
  Product_3f2d6 : Product
  Product_694eb : Product
  Product_910d6 : Product
  Product_9c748 : Product
  Subtract_424f6 : Sum  Inputs=+-
  Blockout_d_id_line_2_3_6d07a : Outport
  wires:
  State_vd_bus_2_5855d/1 -> Product_910d6/2
  Constant_-89.482308708704_658cd/1 -> Product_3f2d6/1
  Product_910d6/1 -> Add_ba6b5/2
  Constant_1904.28407552041_cec53/1 -> Product_910d6/1
  Product_3f2d6/1 -> Add_6ef66/1
  Subtract_424f6/1 -> Blockout_d_id_line_2_3_6d07a/1
  State_id_line_2_3_bbe6e/1 -> Product_3f2d6/2
  Constant_376.991118430775_7f626/1 -> Product_9c748/1
  Product_9c748/1 -> Add_6ef66/2
  State_iq_line_2_3_6cbab/1 -> Product_9c748/2
  Add_6ef66/1 -> Add_ba6b5/1
  Constant_1904.28407552041_4ffae/1 -> Product_694eb/1
  State_vd_bus_3_a3e95/1 -> Product_694eb/2
  Add_ba6b5/1 -> Subtract_424f6/1
  Product_694eb/1 -> Subtract_424f6/2

== system IEEE14_case/AC_1/d_id_line_2_4_block ==
  note: d_id_line_2_4 in case14gfl
      | $376.991118430775\,\mathrm{iq}_{\mathrm{line},2,4}-124.245428153428\,\mathrm{id}_{\mathrm{line},2,4}+2138.10752286057\,\mathrm{vd}_{\mathrm{bus},2}-2138.10752286057\,\mathrm{vd}_{\mathrm{bus},4}$
      | Automatically generated on 2025-10-09 21:39:17 .
  State_id_line_2_4_e6465 : Inport
  State_iq_line_2_4_3e60f : Inport  Port=2
  State_vd_bus_2_934b9 : Inport  Port=3
  State_vd_bus_4_3c016 : Inport  Port=4
  Add_6727a : Sum
  Add_d3d66 : Sum
  Constant_-124.245428153428_e1374 : Constant  Value=-124.245428153428
  Constant_2138.10752286057_29016 : Constant  Value=2138.10752286057
  Constant_2138.10752286057_a35fc : Constant  Value=2138.10752286057
  Constant_376.991118430775_b25da : Constant  Value=376.991118430775
  Product_4796c : Product
  Product_91987 : Product
  Product_a48c6 : Product
  Product_f7818 : Product
  Subtract_e8c08 : Sum  Inputs=+-
  Blockout_d_id_line_2_4_3a4a6 : Outport
  wires:
  Constant_-124.245428153428_e1374/1 -> Product_f7818/1
  Product_a48c6/1 -> Add_6727a/2
  Product_f7818/1 -> Add_6727a/1
  State_id_line_2_4_e6465/1 -> Product_f7818/2
  Constant_376.991118430775_b25da/1 -> Product_a48c6/1
  State_iq_line_2_4_3e60f/1 -> Product_a48c6/2
  Product_4796c/1 -> Add_d3d66/2
  Constant_2138.10752286057_29016/1 -> Product_4796c/1
  State_vd_bus_2_934b9/1 -> Product_4796c/2
  Add_6727a/1 -> Add_d3d66/1
  Product_91987/1 -> Subtract_e8c08/2
  Constant_2138.10752286057_a35fc/1 -> Product_91987/1
  State_vd_bus_4_3c016/1 -> Product_91987/2
  Add_d3d66/1 -> Subtract_e8c08/1
  Subtract_e8c08/1 -> Blockout_d_id_line_2_4_3a4a6/1

== system IEEE14_case/AC_1/d_id_line_2_5_block ==
  note: d_id_line_2_5 in case14gfl
      | $376.991118430775\,\mathrm{iq}_{\mathrm{line},2,5}-123.473914162829\,\mathrm{id}_{\mathrm{line},2,5}+2168.11087204265\,\mathrm{vd}_{\mathrm{bus},2}-2168.11087204265\,\mathrm{vd}_{\mathrm{bus},5}$
      | Automatically generated on 2025-10-09 21:39:19 .
  State_id_line_2_5_d145b : Inport
  State_iq_line_2_5_b0efa : Inport  Port=2
  State_vd_bus_2_cba5a : Inport  Port=3
  State_vd_bus_5_c8ea7 : Inport  Port=4
  Add_cda04 : Sum
  Add_f6f49 : Sum
  Constant_-123.473914162829_f0f2b : Constant  Value=-123.473914162829
  Constant_2168.11087204265_28918 : Constant  Value=2168.11087204265
  Constant_2168.11087204265_4d313 : Constant  Value=2168.11087204265
  Constant_376.991118430775_a3275 : Constant  Value=376.991118430775
  Product_38fe5 : Product
  Product_63be2 : Product
  Product_a9700 : Product
  Product_ac539 : Product
  Subtract_bae2b : Sum  Inputs=+-
  Blockout_d_id_line_2_5_7bd8a : Outport
  wires:
  Constant_-123.473914162829_f0f2b/1 -> Product_38fe5/1
  Constant_376.991118430775_a3275/1 -> Product_63be2/1
  Product_63be2/1 -> Add_cda04/2
  State_id_line_2_5_d145b/1 -> Product_38fe5/2
  State_iq_line_2_5_b0efa/1 -> Product_63be2/2
  Product_ac539/1 -> Add_f6f49/2
  Constant_2168.11087204265_4d313/1 -> Product_ac539/1
  Product_38fe5/1 -> Add_cda04/1
  State_vd_bus_2_cba5a/1 -> Product_ac539/2
  Add_cda04/1 -> Add_f6f49/1
  Product_a9700/1 -> Subtract_bae2b/2
  Constant_2168.11087204265_28918/1 -> Product_a9700/1
  Add_f6f49/1 -> Subtract_bae2b/1
  State_vd_bus_5_c8ea7/1 -> Product_a9700/2
  Subtract_bae2b/1 -> Blockout_d_id_line_2_5_7bd8a/1

== system IEEE14_case/AC_1/d_id_line_3_4_block ==
  note: d_id_line_3_4 in case14gfl
      | $376.991118430775\,\mathrm{iq}_{\mathrm{line},3,4}-147.706103292091\,\mathrm{id}_{\mathrm{line},3,4}+2204.23971484988\,\mathrm{vd}_{\mathrm{bus},3}-2204.23971484988\,\mathrm{vd}_{\mathrm{bus},4}$
      | Automatically generated on 2025-10-09 21:39:21 .
  State_id_line_3_4_8ed23 : Inport
  State_iq_line_3_4_6988a : Inport  Port=2
  State_vd_bus_3_4e043 : Inport  Port=3
  State_vd_bus_4_4b57b : Inport  Port=4
  Add_6dd03 : Sum
  Add_b0ea3 : Sum
  Constant_-147.706103292091_270b7 : Constant  Value=-147.706103292091
  Constant_2204.23971484988_3b171 : Constant  Value=2204.23971484988
  Constant_2204.23971484988_dfc2a : Constant  Value=2204.23971484988
  Constant_376.991118430775_8c9fc : Constant  Value=376.991118430775
  Product_14676 : Product
  Product_5d74e : Product
  Product_db667 : Product
  Product_e8144 : Product
  Subtract_6a90e : Sum  Inputs=+-
  Blockout_d_id_line_3_4_73a35 : Outport
  wires:
  Product_14676/1 -> Add_6dd03/1
  Constant_-147.706103292091_270b7/1 -> Product_14676/1
  Subtract_6a90e/1 -> Blockout_d_id_line_3_4_73a35/1
  State_id_line_3_4_8ed23/1 -> Product_14676/2
  Constant_376.991118430775_8c9fc/1 -> Product_5d74e/1
  Product_5d74e/1 -> Add_6dd03/2
  State_iq_line_3_4_6988a/1 -> Product_5d74e/2
  Add_6dd03/1 -> Add_b0ea3/1
  Constant_2204.23971484988_dfc2a/1 -> Product_e8144/1
  State_vd_bus_3_4e043/1 -> Product_e8144/2
  Product_e8144/1 -> Add_b0ea3/2
  Product_db667/1 -> Subtract_6a90e/2
  Constant_2204.23971484988_3b171/1 -> Product_db667/1
  State_vd_bus_4_4b57b/1 -> Product_db667/2
  Add_b0ea3/1 -> Subtract_6a90e/1

== system IEEE14_case/AC_1/d_id_line_4_5_block ==
  note: d_id_line_4_5 in case14gfl
      | $376.991118430775\,\mathrm{iq}_{\mathrm{line},4,5}-119.516300903606\,\mathrm{id}_{\mathrm{line},4,5}+8952.53190289183\,\mathrm{vd}_{\mathrm{bus},4}-8952.53190289183\,\mathrm{vd}_{\mathrm{bus},5}$
      | Automatically generated on 2025-10-09 21:39:23 .
  State_id_line_4_5_a3d02 : Inport
  State_iq_line_4_5_5f8a8 : Inport  Port=2
  State_vd_bus_4_6b1ed : Inport  Port=3
  State_vd_bus_5_24735 : Inport  Port=4
  Add_61b9e : Sum
  Add_ddae4 : Sum
  Constant_-119.516300903606_d560c : Constant  Value=-119.516300903606
  Constant_376.991118430775_f8101 : Constant  Value=376.991118430775
  Constant_8952.53190289183_1565c : Constant  Value=8952.53190289183
  Constant_8952.53190289183_f8447 : Constant  Value=8952.53190289183
  Product_48efa : Product
  Product_90f27 : Product
  Product_ba622 : Product
  Product_be35c : Product
  Subtract_30367 : Sum  Inputs=+-
  Blockout_d_id_line_4_5_bb2ec : Outport
  wires:
  Constant_-119.516300903606_d560c/1 -> Product_be35c/1
  Constant_8952.53190289183_f8447/1 -> Product_48efa/1
  Product_be35c/1 -> Add_ddae4/1
  State_id_line_4_5_a3d02/1 -> Product_be35c/2
  Constant_376.991118430775_f8101/1 -> Product_ba622/1
  Product_ba622/1 -> Add_ddae4/2
  Product_90f27/1 -> Add_61b9e/2
  Constant_8952.53190289183_1565c/1 -> Product_90f27/1
  State_iq_line_4_5_5f8a8/1 -> Product_ba622/2
  State_vd_bus_4_6b1ed/1 -> Product_90f27/2
  Add_ddae4/1 -> Add_61b9e/1
  State_vd_bus_5_24735/1 -> Product_48efa/2
  Add_61b9e/1 -> Subtract_30367/1
  Product_48efa/1 -> Subtract_30367/2
  Subtract_30367/1 -> Blockout_d_id_line_4_5_bb2ec/1

== system IEEE14_case/AC_1/d_id_line_4_7_block ==
  note: d_id_line_4_7 in case14gfl
      | $376.991118430775\,\mathrm{iq}_{\mathrm{line},4,7}+1843.30284639447\,\mathrm{vd}_{\mathrm{bus},4}-1843.30284639447\,\mathrm{vd}_{\mathrm{bus},7}$
      | Automatically generated on 2025-10-09 21:39:25 .
  State_iq_line_4_7_27056 : Inport
  State_vd_bus_4_7fac7 : Inport  Port=2
  State_vd_bus_7_4017f : Inport  Port=3
  Add_7a611 : Sum
  Constant_1843.30284639447_031c0 : Constant  Value=1843.30284639447
  Constant_1843.30284639447_38c17 : Constant  Value=1843.30284639447
  Constant_376.991118430775_bcde1 : Constant  Value=376.991118430775
  Product_3c801 : Product
  Product_bf7cf : Product
  Product_c16bb : Product
  Subtract_86085 : Sum  Inputs=+-
  Blockout_d_id_line_4_7_734b6 : Outport
  wires:
  State_vd_bus_7_4017f/1 -> Product_3c801/2
  Product_c16bb/1 -> Add_7a611/1
  Constant_376.991118430775_bcde1/1 -> Product_c16bb/1
  State_iq_line_4_7_27056/1 -> Product_c16bb/2
  Constant_1843.30284639447_031c0/1 -> Product_bf7cf/1
  Product_bf7cf/1 -> Add_7a611/2
  State_vd_bus_4_7fac7/1 -> Product_bf7cf/2
  Constant_1843.30284639447_38c17/1 -> Product_3c801/1
  Add_7a611/1 -> Subtract_86085/1
  Product_3c801/1 -> Subtract_86085/2
  Subtract_86085/1 -> Blockout_d_id_line_4_7_734b6/1

== system IEEE14_case/AC_1/d_id_line_4_9_block ==
  note: d_id_line_4_9 in case14gfl
      | $376.991118430775\,\mathrm{iq}_{\mathrm{line},4,9}+699.506853548825\,\mathrm{vd}_{\mathrm{bus},4}-699.506853548825\,\mathrm{vd}_{\mathrm{bus},9}$
      | Automatically generated on 2025-10-09 21:39:27 .
  State_iq_line_4_9_4287b : Inport
  State_vd_bus_4_34e3c : Inport  Port=2
  State_vd_bus_9_e9340 : Inport  Port=3
  Add_9883b : Sum
  Constant_376.991118430775_a95c9 : Constant  Value=376.991118430775
  Constant_699.506853548825_c1268 : Constant  Value=699.506853548825
  Constant_699.506853548825_ef2c8 : Constant  Value=699.506853548825
  Product_a1bfd : Product
  Product_a2d56 : Product
  Product_c75a4 : Product
  Subtract_e39d7 : Sum  Inputs=+-
  Blockout_d_id_line_4_9_c5562 : Outport
  wires:
  Constant_376.991118430775_a95c9/1 -> Product_c75a4/1
  State_iq_line_4_9_4287b/1 -> Product_c75a4/2
  Constant_699.506853548825_ef2c8/1 -> Product_a2d56/1
  Product_a2d56/1 -> Add_9883b/2
  State_vd_bus_4_34e3c/1 -> Product_a2d56/2
  Product_c75a4/1 -> Add_9883b/1
  Constant_699.506853548825_c1268/1 -> Product_a1bfd/1
  Product_a1bfd/1 -> Subtract_e39d7/2
  State_vd_bus_9_e9340/1 -> Product_a1bfd/2
  Add_9883b/1 -> Subtract_e39d7/1
  Subtract_e39d7/1 -> Blockout_d_id_line_4_9_c5562/1

== system IEEE14_case/AC_1/d_id_line_5_6_block ==
  note: d_id_line_5_6 in case14gfl
      | $376.991118430775\,\mathrm{iq}_{\mathrm{line},5,6}+1605.01907859506\,\mathrm{vd}_{\mathrm{bus},5}-1605.01907859506\,\mathrm{vd}_{\mathrm{bus},6}$
      | Automatically generated on 2025-10-09 21:39:29 .
  State_iq_line_5_6_d8c49 : Inport
  State_vd_bus_5_45df8 : Inport  Port=2
  State_vd_bus_6_a8e09 : Inport  Port=3
  Add_a44a6 : Sum
  Constant_1605.01907859506_4e22b : Constant  Value=1605.01907859506
  Constant_1605.01907859506_6f317 : Constant  Value=1605.01907859506
  Constant_376.991118430775_1a51a : Constant  Value=376.991118430775
  Product_3c99a : Product
  Product_4e7f7 : Product
  Product_55d32 : Product
  Subtract_9cfda : Sum  Inputs=+-
  Blockout_d_id_line_5_6_7c54f : Outport
  wires:
  State_vd_bus_6_a8e09/1 -> Product_55d32/2
  Add_a44a6/1 -> Subtract_9cfda/1
  Constant_376.991118430775_1a51a/1 -> Product_4e7f7/1
  Constant_1605.01907859506_4e22b/1 -> Product_55d32/1
  State_iq_line_5_6_d8c49/1 -> Product_4e7f7/2
  Constant_1605.01907859506_6f317/1 -> Product_3c99a/1
  Product_3c99a/1 -> Add_a44a6/2
  State_vd_bus_5_45df8/1 -> Product_3c99a/2
  Product_4e7f7/1 -> Add_a44a6/1
  Product_55d32/1 -> Subtract_9cfda/2
  Subtract_9cfda/1 -> Blockout_d_id_line_5_6_7c54f/1

== system IEEE14_case/AC_1/d_id_line_6_11_block ==
  note: d_id_line_6_11 in case14gfl
      | $376.991118430775\,\mathrm{iq}_{\mathrm{line},6,11}-180.023209796657\,\mathrm{id}_{\mathrm{line},6,11}+1895.38018316126\,\mathrm{vd}_{\mathrm{bus},6}-1895.38018316126\,\mathrm{vd}_{\mathrm{bus},11}$
      | Automatically generated on 2025-10-09 21:39:31 .
  State_id_line_6_11_a0eef : Inport
  State_iq_line_6_11_43c10 : Inport  Port=2
  State_vd_bus_11_0f741 : Inport  Port=3
  State_vd_bus_6_98960 : Inport  Port=4
  Add_ca7f5 : Sum
  Add_e5739 : Sum
  Constant_-180.023209796657_43956 : Constant  Value=-180.023209796657
  Constant_1895.38018316126_4e0bb : Constant  Value=1895.38018316126
  Constant_1895.38018316126_5b54e : Constant  Value=1895.38018316126
  Constant_376.991118430775_e0f6a : Constant  Value=376.991118430775
  Product_3aa25 : Product
  Product_640c9 : Product
  Product_8816d : Product
  Product_c21c0 : Product
  Subtract_d09fb : Sum  Inputs=+-
  Blockout_d_id_line_6_11_26563 : Outport
  wires:
  Constant_-180.023209796657_43956/1 -> Product_640c9/1
  Product_640c9/1 -> Add_e5739/1
  Product_c21c0/1 -> Add_e5739/2
  State_id_line_6_11_a0eef/1 -> Product_640c9/2
  Subtract_d09fb/1 -> Add_ca7f5/1
  Constant_376.991118430775_e0f6a/1 -> Product_c21c0/1
  State_iq_line_6_11_43c10/1 -> Product_c21c0/2
  Product_8816d/1 -> Subtract_d09fb/2
  Constant_1895.38018316126_5b54e/1 -> Product_8816d/1
  Add_ca7f5/1 -> Blockout_d_id_line_6_11_26563/1
  State_vd_bus_11_0f741/1 -> Product_8816d/2
  Add_e5739/1 -> Subtract_d09fb/1
  Product_3aa25/1 -> Add_ca7f5/2
  Constant_1895.38018316126_4e0bb/1 -> Product_3aa25/1
  State_vd_bus_6_98960/1 -> Product_3aa25/2

== system IEEE14_case/AC_1/d_id_line_6_12_block ==
  note: d_id_line_6_12 in case14gfl
      | $376.991118430775\,\mathrm{iq}_{\mathrm{line},6,12}-181.134351144703\,\mathrm{id}_{\mathrm{line},6,12}+1473.7153294663\,\mathrm{vd}_{\mathrm{bus},6}-1473.7153294663\,\mathrm{vd}_{\mathrm{bus},12}$
      | Automatically generated on 2025-10-09 21:39:33 .
  State_id_line_6_12_9e271 : Inport
  State_iq_line_6_12_68573 : Inport  Port=2
  State_vd_bus_12_ff782 : Inport  Port=3
  State_vd_bus_6_ffde5 : Inport  Port=4
  Add_75c9f : Sum
  Add_bd310 : Sum
  Constant_-181.134351144703_e8bb4 : Constant  Value=-181.134351144703
  Constant_1473.7153294663_18c13 : Constant  Value=1473.7153294663
  Constant_1473.7153294663_37410 : Constant  Value=1473.7153294663
  Constant_376.991118430775_4a305 : Constant  Value=376.991118430775
  Product_0a75c : Product
  Product_441f2 : Product
  Product_b24e8 : Product
  Product_dba87 : Product
  Subtract_e78a4 : Sum  Inputs=+-
  Blockout_d_id_line_6_12_9a391 : Outport
  wires:
  Constant_-181.134351144703_e8bb4/1 -> Product_0a75c/1
  State_id_line_6_12_9e271/1 -> Product_0a75c/2
  Constant_376.991118430775_4a305/1 -> Product_dba87/1
  Product_dba87/1 -> Add_75c9f/2
  State_iq_line_6_12_68573/1 -> Product_dba87/2
  Product_0a75c/1 -> Add_75c9f/1
  State_vd_bus_12_ff782/1 -> Product_441f2/2
  Product_441f2/1 -> Subtract_e78a4/2
  Constant_1473.7153294663_37410/1 -> Product_441f2/1
  Add_75c9f/1 -> Subtract_e78a4/1
  Product_b24e8/1 -> Add_bd310/2
  Constant_1473.7153294663_18c13/1 -> Product_b24e8/1
  State_vd_bus_6_ffde5/1 -> Product_b24e8/2
  Subtract_e78a4/1 -> Add_bd310/1
  Add_bd310/1 -> Blockout_d_id_line_6_12_9a391/1

== system IEEE14_case/AC_1/d_id_line_6_13_block ==
  note: d_id_line_6_13 in case14gfl
      | $376.991118430775\,\mathrm{iq}_{\mathrm{line},6,13}-191.432889262269\,\mathrm{id}_{\mathrm{line},6,13}+2893.92122845456\,\mathrm{vd}_{\mathrm{bus},6}-2893.92122845456\,\mathrm{vd}_{\mathrm{bus},13}$
      | Automatically generated on 2025-10-09 21:39:35 .
  State_id_line_6_13_e3fb9 : Inport
  State_iq_line_6_13_c66be : Inport  Port=2
  State_vd_bus_13_13060 : Inport  Port=3
  State_vd_bus_6_845eb : Inport  Port=4
  Add_04197 : Sum
  Add_871b2 : Sum
  Constant_-191.432889262269_1e554 : Constant  Value=-191.432889262269
  Constant_2893.92122845456_3f8a7 : Constant  Value=2893.92122845456
  Constant_2893.92122845456_64313 : Constant  Value=2893.92122845456
  Constant_376.991118430775_c04fb : Constant  Value=376.991118430775
  Product_530db : Product
  Product_67b5d : Product
  Product_84309 : Product
  Product_c3918 : Product
  Subtract_aac24 : Sum  Inputs=+-
  Blockout_d_id_line_6_13_cc035 : Outport
  wires:
  State_vd_bus_13_13060/1 -> Product_530db/2
  Constant_-191.432889262269_1e554/1 -> Product_84309/1
  Constant_2893.92122845456_64313/1 -> Product_530db/1
  Add_871b2/1 -> Blockout_d_id_line_6_13_cc035/1
  State_id_line_6_13_e3fb9/1 -> Product_84309/2
  Constant_376.991118430775_c04fb/1 -> Product_67b5d/1
  Product_67b5d/1 -> Add_04197/2
  State_iq_line_6_13_c66be/1 -> Product_67b5d/2
  Product_84309/1 -> Add_04197/1
  Add_04197/1 -> Subtract_aac24/1
  Product_530db/1 -> Subtract_aac24/2
  Product_c3918/1 -> Add_871b2/2
  Constant_2893.92122845456_3f8a7/1 -> Product_c3918/1
  State_vd_bus_6_845eb/1 -> Product_c3918/2
  Subtract_aac24/1 -> Add_871b2/1

== system IEEE14_case/AC_1/d_id_line_7_8_block ==
  note: d_id_line_7_8 in case14gfl
      | $376.991118430775\,\mathrm{iq}_{\mathrm{line},7,8}+2140.17098172453\,\mathrm{vd}_{\mathrm{bus},7}-2140.17098172453\,\mathrm{vd}_{\mathrm{bus},8}$
      | Automatically generated on 2025-10-09 21:39:37 .
  State_iq_line_7_8_7266b : Inport
  State_vd_bus_7_8b12e : Inport  Port=2
  State_vd_bus_8_dd54f : Inport  Port=3
  Add_7a258 : Sum
  Constant_2140.17098172453_75291 : Constant  Value=2140.17098172453
  Constant_2140.17098172453_aac7d : Constant  Value=2140.17098172453
  Constant_376.991118430775_8ae43 : Constant  Value=376.991118430775
  Product_262f2 : Product
  Product_a35d8 : Product
  Product_c394f : Product
  Subtract_bdc88 : Sum  Inputs=+-
  Blockout_d_id_line_7_8_3aa11 : Outport
  wires:
  Product_c394f/1 -> Add_7a258/1
  Constant_376.991118430775_8ae43/1 -> Product_c394f/1
  Constant_2140.17098172453_75291/1 -> Product_262f2/1
  Product_262f2/1 -> Add_7a258/2
  State_iq_line_7_8_7266b/1 -> Product_c394f/2
  State_vd_bus_7_8b12e/1 -> Product_262f2/2
  Product_a35d8/1 -> Subtract_bdc88/2
  Constant_2140.17098172453_aac7d/1 -> Product_a35d8/1
  State_vd_bus_8_dd54f/1 -> Product_a35d8/2
  Add_7a258/1 -> Subtract_bdc88/1
  Subtract_bdc88/1 -> Blockout_d_id_line_7_8_3aa11/1
